simulink model "StateSpaceControllerNominal"  (R2020b)
settings: Solver=ode45  StartTime=0.0  StopTime=10.0  MaxStep=0.001  RelTol=1e-3
settings Model: Creator=umberto  LastModifiedBy=umberto

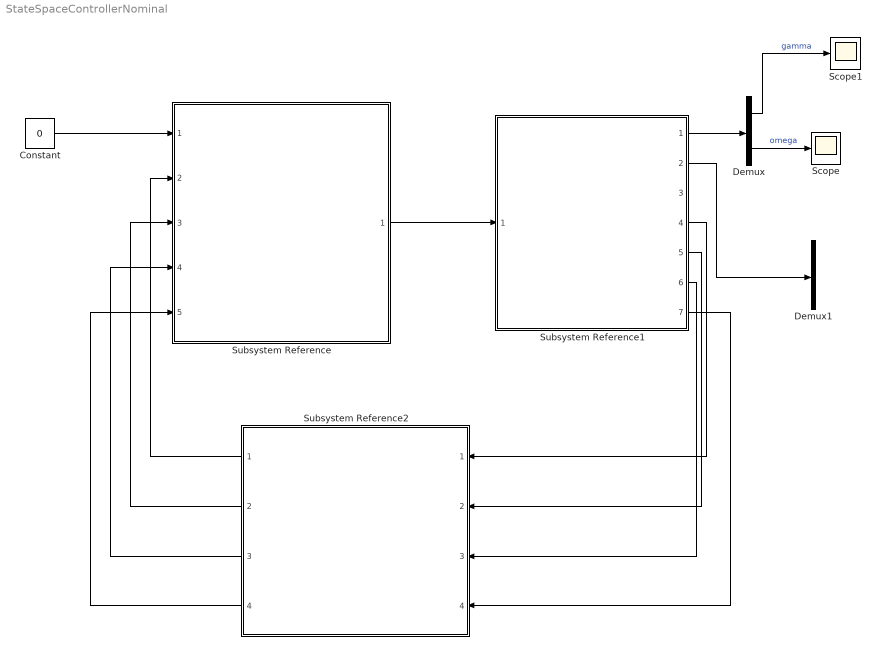
== system StateSpaceControllerNominal ==
  Constant : Constant  Value=0
  Demux : Demux  Outputs=2
  Demux1 : Demux  Outputs=2
  Scope : Scope
  Scope1 : Scope
  Subsystem Reference : Subsystem  ReferencedSubsystem=StateSpaceControllerNominal_SubSystem
  Subsystem Reference1 : Subsystem  ReferencedSubsystem=Robot_SubSystem
  Subsystem Reference2 : Subsystem  ReferencedSubsystem=SimpleStateObserver_SubSystem
  wires:
  Subsystem Reference1/4 -> Subsystem Reference2/1
  Subsystem Reference1/5 -> Subsystem Reference2/2
  Subsystem Reference1/6 -> Subsystem Reference2/3
  Subsystem Reference1/7 -> Subsystem Reference2/4
  Subsystem Reference2/1 -> Subsystem Reference/2
  Subsystem Reference2/2 -> Subsystem Reference/3
  Subsystem Reference2/3 -> Subsystem Reference/4
  Subsystem Reference2/4 -> Subsystem Reference/5
  Subsystem Reference/1 -> Subsystem Reference1/1
  Subsystem Reference1/1 -> Demux/1
  Demux/2 -> Scope/1  "omega"
  Demux/1 -> Scope1/1  "gamma"
  Constant/1 -> Subsystem Reference/1
  Subsystem Reference1/2 -> Demux1/1
